simulink model "w2p2"  (R2020b)
settings: Solver=VariableStepAuto  StartTime=0.0  StopTime=10.0  RelTol=1e-3
values from neighbouring files (symbols this model uses):
  be = 2.0    [data_dict.sldd]
  bv = 1.0    [data_dict.sldd]
  Ie = 1.0    [data_dict.sldd]
  Iv = 5.0    [data_dict.sldd]
settings Model: Creator=Dell  LastModifiedBy=Dell

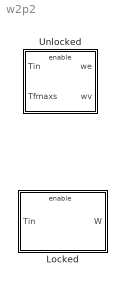
== system w2p2 ==
  Locked : Subsystem
  Unlocked : Subsystem

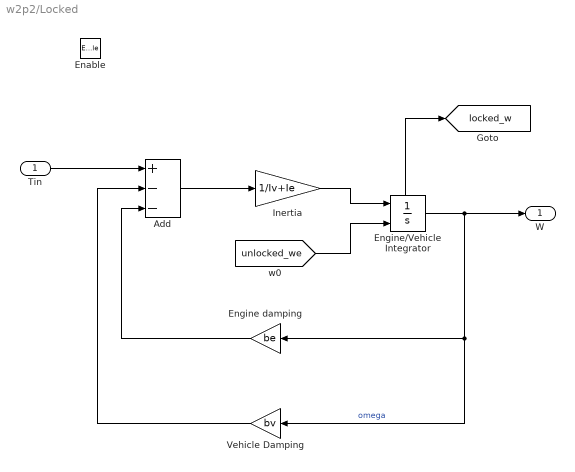
== system w2p2/Locked ==
  Tin : Inport
  Enable : EnablePort
  Add : Sum  Inputs=+--
  Engine damping : Gain  Gain=be
  Engine/Vehicle Integrator : Integrator  InitialConditionSource=external  ShowStatePort=on
  Inertia : Gain  Gain=1/Iv+Ie
  Vehicle Damping : Gain  Gain=bv
  W : Outport
  tag scope: locked_w=global
  wires:
  Add/1 -> Inertia/1
  Engine/Vehicle Integrator/State -> [locked_w]
  [unlocked_we] -> Engine/Vehicle Integrator/2
  Tin/1 -> Add/1
  Vehicle Damping/1 -> Add/2
  Inertia/1 -> Engine/Vehicle Integrator/1
  Engine/Vehicle Integrator/1 -> W/1, Vehicle Damping/1, Engine damping/1  "omega"
  Engine damping/1 -> Add/3

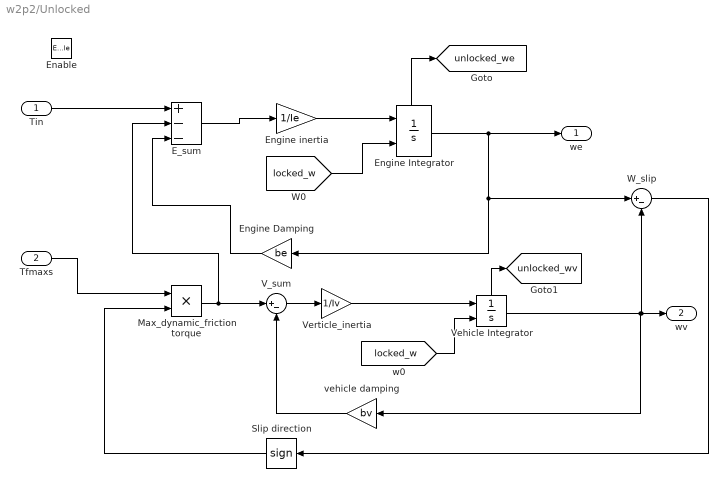
== system w2p2/Unlocked ==
  Tin : Inport
  Tfmaxs : Inport  Port=2
  Enable : EnablePort
  E_sum : Sum  Inputs=+--
  Engine Damping : Gain  Gain=be
  Engine Integrator : Integrator  InitialConditionSource=external  ShowStatePort=on
  Engine inertia : Gain  Gain=1/Ie
  Max_dynamic_friction torque : Product
  Slip direction : Signum
  V_sum : Sum  Inputs=|+-
  Vehicle Integrator : Integrator  InitialConditionSource=external  ShowStatePort=on
  Verticle_inertia : Gain  Gain=1/Iv
  W_slip : Sum  Inputs=|+-
  vehicle damping : Gain  Gain=bv
  we : Outport
  wv : Outport  Port=2
  tag scope: unlocked_we=global, unlocked_wv=global
  wires:
  E_sum/1 -> Engine inertia/1
  Engine Integrator/1 -> Engine Damping/1, W_slip/1, we/1
  Tfmaxs/1 -> Max_dynamic_friction torque/1
  Slip direction/1 -> Max_dynamic_friction torque/2
  [locked_w] -> Engine Integrator/2
  V_sum/1 -> Verticle_inertia/1
  Vehicle Integrator/1 -> wv/1, W_slip/2, vehicle damping/1
  Engine inertia/1 -> Engine Integrator/1
  Max_dynamic_friction torque/1 -> V_sum/1, E_sum/2
  W_slip/1 -> Slip direction/1
  Vehicle Integrator/State -> [unlocked_wv]
  Verticle_inertia/1 -> Vehicle Integrator/1
  [locked_w] -> Vehicle Integrator/2
  Engine Integrator/State -> [unlocked_we]
  Tin/1 -> E_sum/1
  Engine Damping/1 -> E_sum/3
  vehicle damping/1 -> V_sum/2
